simulink model "Test_fuzzy_logic_offline"  (R2020b)
settings: Solver=VariableStepAuto  StartTime=0.0  StopTime=13.5  RelTol=1e-3
undefined symbols (not defined in the file or in its folder): theta_dot_5
libraries: fuzblock x1
settings Model: Creator=Mario Faragalla  LastModifiedBy=Mario Faragalla

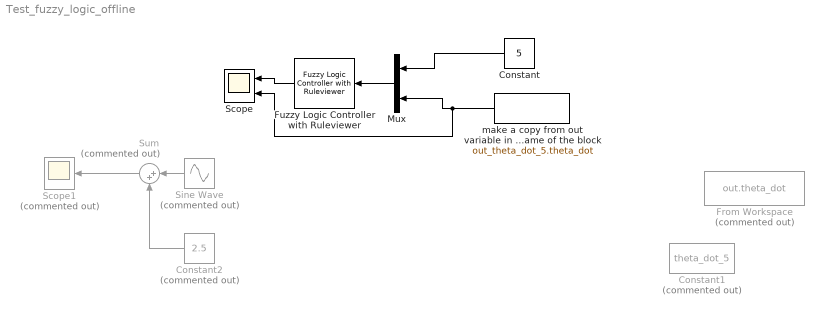
== system Test_fuzzy_logic_offline ==
  Constant : Constant  Value=5
  Constant1 : Constant  Commented=on  Value=theta_dot_5
  Constant2 : Constant  Commented=on  Value=2.5
  From Workspace : FromWorkspace  Commented=on  VariableName=out.theta_dot
  Fuzzy Logic Controller with Ruleviewer : fuzblock/Fuzzy Logic  Controller  with Ruleviewer  fismatrix=fuzzy_pile3  Ts=2
  Mux : Mux  Inputs=2
  Scope : Scope  NumInputPorts=2
  Scope1 : Scope  Commented=on
  Sine Wave : Sin  Commented=on  Amplitude=2.5  Frequency=0.25  SampleTime=0
  Sum : Sum  Commented=on  Inputs=|++
  make a copy from out variable in the other file to the workspace then rename it with the name of the block : FromWorkspace  VariableName=out_theta_dot_5.theta_dot
  wires:
  Mux/1 -> Fuzzy Logic Controller with Ruleviewer/1
  Constant/1 -> Mux/1
  make a copy from out variable in the other file to the workspace then rename it with the name of the block/1 -> Scope/2, Mux/2
  Fuzzy Logic Controller with Ruleviewer/1 -> Scope/1
  Sine Wave/1 -> Sum/1
  Constant2/1 -> Sum/2
  Sum/1 -> Scope1/1
